simulink model "PDS"  (R2023a)
settings: Solver=VariableStepAuto  StartTime=0.0  StopTime=5  RelTol=1e-3
settings Model: Creator=DELL  LastModifiedBy=DELL

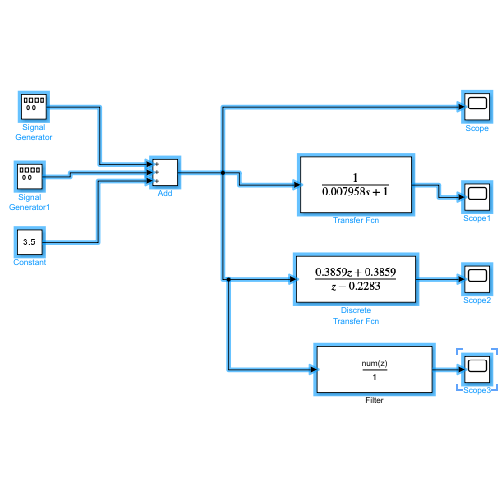
[thumbnail: Simulink's stored preview of the top-level diagram]
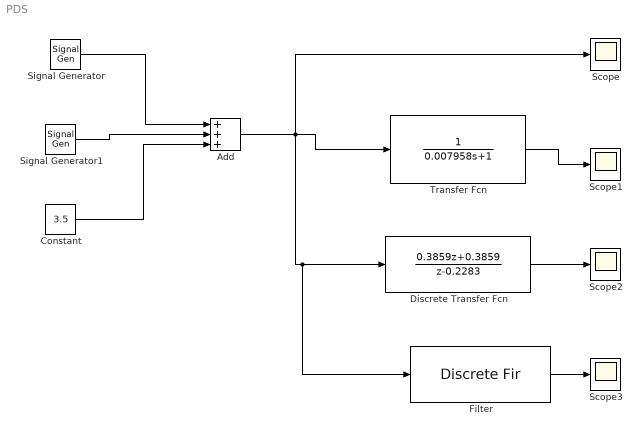
== system PDS ==
  Add : Sum  Inputs=+++
  Constant : Constant  Value=3.5
  Discrete Transfer Fcn : DiscreteTransferFcn  Numerator=[0.3859 0.3859]  Denominator=[1 -0.2283]  SampleTime=0.01
  Filter : DiscreteFir  Tag=BlockMethodSubSystem  Coefficients=[0 0.0184617817076260203 0.0680541696671083801 0.130643334905041958 0.18197961203066973 0.201722203379107984 0.18197961203066973 0.130643334905041958 0.0680541696671083801 0.0184617817076260203 0]  InputProcessing=Columns as channels (frame based)
  Scope{,1..3} (4 alike) : Scope
  Signal Generator : SignalGenerator  Amplitude=3
  Signal Generator1 : SignalGenerator  Amplitude=0.4  Frequency=100
  Transfer Fcn : TransferFcn  Denominator=[0.007958 1]
  wires:
  Signal Generator/1 -> Add/1
  Constant/1 -> Add/3
  Signal Generator1/1 -> Add/2
  Add/1 -> Filter/1, Discrete Transfer Fcn/1, Scope/1, Transfer Fcn/1
  Transfer Fcn/1 -> Scope1/1
  Discrete Transfer Fcn/1 -> Scope2/1
  Filter/1 -> Scope3/1
